simulink model "Simulink"  (R2024b)
settings: Solver=FixedStepAuto  StartTime=0.0  StopTime=tf_sim  FixedStep=dt/time_scale  MaxStep=dt/100  RelTol=1e-3
values from neighbouring files (symbols this model uses):
  A_ref = zeros(nx,nx,N_ref)    [Main.m]
  b_bar = repmat(b_tilde,N,1)    [Main.m]
  B_ref = zeros(nx,nu,N_ref)    [Main.m]
  d = 0.1    [Main.m]
  dt = tf_ref/N_ref    [Main.m]
  H_ter = terminalXf.H    [Main.m]
  h_ter = terminalXf.h    [Main.m]
  IC_obs = [IC_obs_state; IC_obs_d]    [Main.m]
  N = 20    [Main.m]
  nu = size(u_ref,2)    [Main.m]
  nx = size(x_ref,2)    [Main.m]
  Q_obs = blkdiag(Qw,Qp)    [Main.m]
  R_obs = diag([1 1 1])    [Main.m]
  time_scale = 1    [Main.m]
  Ub_lb = repmat(u_min,N_ref,1)-Umat2Uvect(u_ref)    [Main.m]
  Ub_ub = repmat(u_max,N_ref,1)-Umat2Uvect(u_ref)    [Main.m]
  v_max = 0.55    [Main.m]
  v_min = 0.2    [Main.m]
  w_max = 1    [Main.m]
  w_min = -1    [Main.m]
undefined symbols (not defined in the file or in its folder): Angular, DiscIntNeverNeededParam, H_sim, h_sim, Linear, S_sim, T_sim
libraries: robotlib x3
settings Model: Creator=nicvi  LastModifiedBy=vise
settings OptimizationCC: DefaultParameterBehavior=Inlined  EnhancedBackFolding=on  PassReuseOutputArgsAs=Individual arguments  ZeroExternalMemoryAtStartup=off  ZeroInternalMemoryAtStartup=off  MaxStackSize=64  OptimizeBlockOrder=speed  DifferentSizesBufferReuse=on  OptimizationCustomize=off  EfficientTunableParamExpr=on
settings DebuggingCC: ParameterTunabilityLossMsg=error
settings HardwareCC: ProdBitPerPointer=32  ProdBitPerSizeT=32  ProdBitPerPtrDiffT=32  ProdLargestAtomicFloat=None  ProdIntDivRoundTo=Undefined  ProdEndianess=Unspecified  ProdWordSize=32  ProdHWDeviceType=Generic->Unspecified (assume 32-bit Generic)  UseEmbeddedCoderFeatures=off
settings RTWCC: Description=Embedded Coder  SystemTargetFile=ert.tlc  HardwareBoard=Robot Operating System (ROS)  TLCOptions="-aInlineSetEventsForThisBaseRateFcn=TLC_FALSE -aSuppressMultiTaskScheduler=TLC_FALSE  -aRateBasedStepFcn=0"  TemplateMakefile=ert_default_tmf  Toolchain=Catkin  TargetLang=C++
settings CodeAppCC: ForceParamTrailComments=on  IgnoreCustomStorageClasses=off  OperatorAnnotations=on  SimulinkDataObjDesc=on  SFDataObjDesc=on  InsertBlockDesc=on
settings ERTTargetCC: SupportNonInlinedSFcns=on

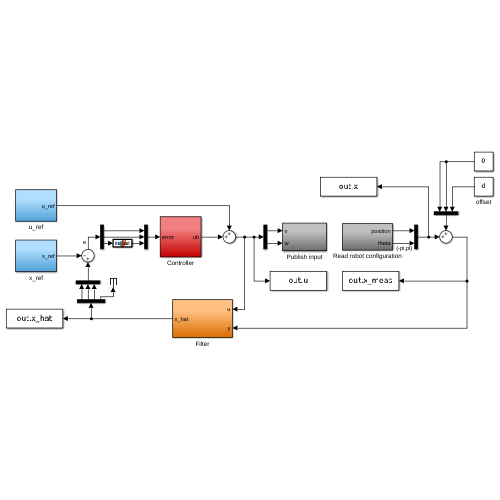
[thumbnail: Simulink's stored preview of the top-level diagram]
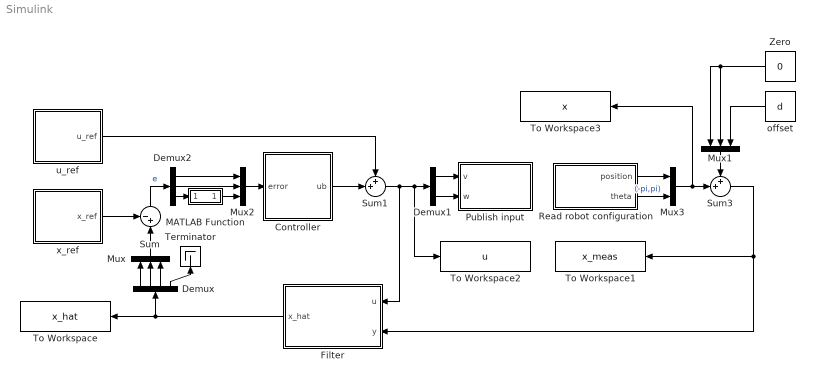
== system Simulink ==
  Controller : Subsystem
  Demux : Demux
  Demux1 : Demux  Outputs=2
  Demux2 : Demux  Outputs=3
  Filter : Subsystem
  MATLAB Function : MATLAB Function  TreatAsAtomicUnit=on
  Mux : Mux  Inputs=3
  Mux1 : Mux  Inputs=3
  Mux2 : Mux  Inputs=3
  Mux3 : Mux  Inputs=2
  Publish input : Subsystem
  Read robot configuration : Subsystem
  Sum : Sum  Inputs=-+|
  Sum1 : Sum  Inputs=++|
  Sum3 : Sum  Inputs=++|
  Terminator : Terminator
  To Workspace : ToWorkspace  VariableName=x_hat  SampleTime=-1
  To Workspace1 : ToWorkspace  VariableName=x_meas  SampleTime=-1
  To Workspace2 : ToWorkspace  VariableName=u  SampleTime=dt/time_scale
  To Workspace3 : ToWorkspace  VariableName=x  SampleTime=-1
  Zero : Constant  Value=0  OutDataTypeStr=Inherit: Inherit via back propagation
  offset : Constant  Value=d
  u_ref : Subsystem
  x_ref : Subsystem
  wires:
  x_ref/1(x_ref) -> Sum/1
  Controller/1(ub) -> Sum1/2
  u_ref/1(u_ref) -> Sum1/1
  Sum/1 -> Demux2/1  "e"
  Sum1/1 -> Filter/1(u), Demux1/1, To Workspace2/1
  Mux3/1 -> To Workspace3/1, Sum3/2
  Filter/1(x_hat) -> To Workspace/1, Demux/1
  Demux/1 -> Mux/1
  Demux/4 -> Terminator/1
  Demux/2 -> Mux/2
  Demux/3 -> Mux/3
  Mux/1 -> Sum/2
  offset/1 -> Mux1/3
  Mux1/1 -> Sum3/1
  Demux2/3 -> MATLAB Function/1(in)
  MATLAB Function/1(out) -> Mux2/3
  Demux2/1 -> Mux2/1
  Demux2/2 -> Mux2/2
  Mux2/1 -> Controller/1(error)
  Zero/1 -> Mux1/1, Mux1/2
  Demux1/1 -> Publish input/1(v)
  Demux1/2 -> Publish input/2(w)
  Read robot configuration/1(position) -> Mux3/1
  Read robot configuration/2(theta) -> Mux3/2  "(-pi,pi)"
  Sum3/1 -> Filter/2(y), To Workspace1/1

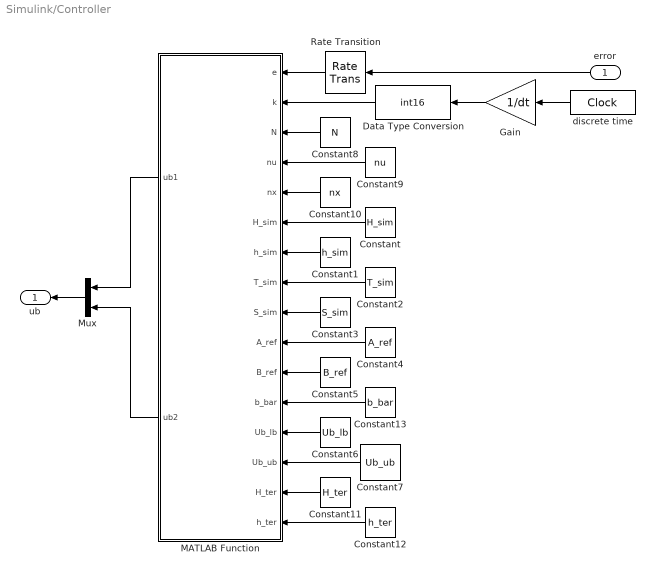
== system Simulink/Controller ==
  error : Inport
  Constant : Constant  Value=H_sim
  Constant1 : Constant  Value=h_sim
  Constant10 : Constant  Value=nx
  Constant11 : Constant  Value=H_ter
  Constant12 : Constant  Value=h_ter
  Constant13 : Constant  Value=b_bar
  Constant2 : Constant  Value=T_sim
  Constant3 : Constant  Value=S_sim
  Constant4 : Constant  Value=A_ref
  Constant5 : Constant  Value=B_ref
  Constant6 : Constant  Value=Ub_lb
  Constant7 : Constant  Value=Ub_ub
  Constant8 : Constant  Value=N
  Constant9 : Constant  Value=nu
  Data Type Conversion : DataTypeConversion  OutDataTypeStr=int16  SaturateOnIntegerOverflow=off  RndMeth=Floor
  Gain : Gain  Gain=1/dt
  MATLAB Function : MATLAB Function  TreatAsAtomicUnit=on
  Mux : Mux  Inputs=2
  Rate Transition : RateTransition  OutPortSampleTime=dt
  discrete time : DigitalClock  SampleTime=dt
  ub : Outport
  wires:
  Constant4/1 -> MATLAB Function/10(A_ref)
  Data Type Conversion/1 -> MATLAB Function/2(k)
  discrete time/1 -> Gain/1
  Gain/1 -> Data Type Conversion/1
  Rate Transition/1 -> MATLAB Function/1(e)
  Constant10/1 -> MATLAB Function/5(nx)
  Constant11/1 -> MATLAB Function/15(H_ter)
  Constant13/1 -> MATLAB Function/12(b_bar)
  Constant5/1 -> MATLAB Function/11(B_ref)
  Constant3/1 -> MATLAB Function/9(S_sim)
  Constant6/1 -> MATLAB Function/13(Ub_lb)
  Constant9/1 -> MATLAB Function/4(nu)
  Constant7/1 -> MATLAB Function/14(Ub_ub)
  Constant12/1 -> MATLAB Function/16(h_ter)
  Constant8/1 -> MATLAB Function/3(N)
  Constant1/1 -> MATLAB Function/7(h_sim)
  Constant2/1 -> MATLAB Function/8(T_sim)
  error/1 -> Rate Transition/1
  MATLAB Function/1(ub1) -> Mux/1
  MATLAB Function/2(ub2) -> Mux/2
  Mux/1 -> ub/1
  Constant/1 -> MATLAB Function/6(H_sim)

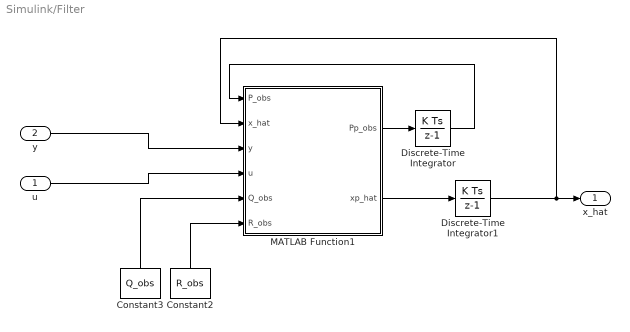
== system Simulink/Filter ==
  u : Inport
  y : Inport  Port=2
  Constant2 : Constant  Value=R_obs
  Constant3 : Constant  Value=Q_obs
  Discrete-Time Integrator : DiscreteIntegrator  InitialCondition=zeros(nx+1,nx+1)  SampleTime=-1  ICPrevOutput=DiscIntNeverNeededParam  ICPrevScaledInput=DiscIntNeverNeededParam
  Discrete-Time Integrator1 : DiscreteIntegrator  InitialCondition=IC_obs  SampleTime=-1  ICPrevOutput=DiscIntNeverNeededParam  ICPrevScaledInput=DiscIntNeverNeededParam
  MATLAB Function1 : MATLAB Function  TreatAsAtomicUnit=on
  x_hat : Outport
  wires:
  MATLAB Function1/1(Pp_obs) -> Discrete-Time Integrator/1
  Constant3/1 -> MATLAB Function1/5(Q_obs)
  Constant2/1 -> MATLAB Function1/6(R_obs)
  Discrete-Time Integrator/1 -> MATLAB Function1/1(P_obs)
  Discrete-Time Integrator1/1 -> x_hat/1, MATLAB Function1/2(x_hat)
  MATLAB Function1/2(xp_hat) -> Discrete-Time Integrator1/1
  y/1 -> MATLAB Function1/3(y)
  u/1 -> MATLAB Function1/4(u)

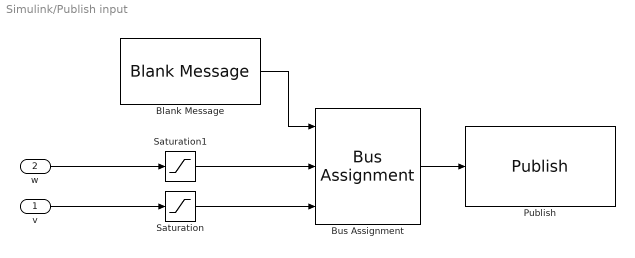
== system Simulink/Publish input ==
  v : Inport
  w : Inport  Port=2
  Blank Message : robotlib/Blank Message  messageClass=Message  entityType=geometry_msgs/Twist  messageType=geometry_msgs/Twist  SampleTime=dt  legacyBusStruct=off
  Bus Assignment : BusAssignment  AssignedSignals=Angular.Z,Linear.X
  Publish : robotlib/Publish  topicSource=Select from ROS network  topic=/cmd_vel  messageType=geometry_msgs/Twist  legacyBusStruct=off  messageQueueLength=1
  Saturation : Saturate  UpperLimit=v_max  LowerLimit=v_min
  Saturation1 : Saturate  UpperLimit=w_max  LowerLimit=w_min
  wires:
  Bus Assignment/1 -> Publish/1
  Blank Message/1 -> Bus Assignment/1
  w/1 -> Saturation1/1
  v/1 -> Saturation/1
  Saturation/1 -> Bus Assignment/3
  Saturation1/1 -> Bus Assignment/2

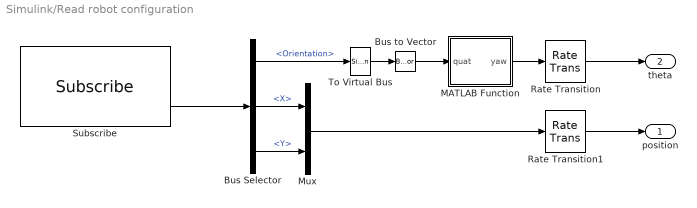
== system Simulink/Read robot configuration ==
  Bus Selector : BusSelector  OutputSignals=Pose.Pose.Orientation,Pose.Pose.Position.X,Pose.Pose.Position.Y
  Bus to Vector : BusToVector
  MATLAB Function : MATLAB Function  TreatAsAtomicUnit=on
  Mux : Mux  Inputs=2
  Rate Transition : RateTransition
  Rate Transition1 : RateTransition
  Subscribe : robotlib/Subscribe  topicSource=Select from ROS network  topic=/odom  messageType=nav_msgs/Odometry  SampleTime=dt  legacyBusStruct=off  messageQueueLength=1
  To Virtual Bus : SignalConversion  ConversionOutput=Virtual bus  OverrideOpt=off
  position : Outport
  theta : Outport  Port=2
  wires:
  Bus to Vector/1 -> MATLAB Function/1(quat)
  Bus Selector/1 -> To Virtual Bus/1  "<Orientation>"
  Bus Selector/2 -> Mux/1  "<X>"
  To Virtual Bus/1 -> Bus to Vector/1
  Subscribe/2 -> Bus Selector/1
  Bus Selector/3 -> Mux/2  "<Y>"
  MATLAB Function/1(yaw) -> Rate Transition/1
  Mux/1 -> Rate Transition1/1
  Rate Transition/1 -> theta/1
  Rate Transition1/1 -> position/1

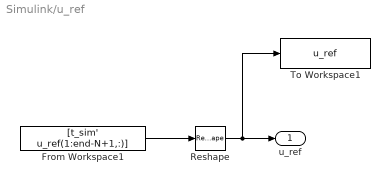
== system Simulink/u_ref ==
  From Workspace1 : FromWorkspace  VariableName="[t_sim'  u_ref(1:end-N+1,:)]"  SampleTime=dt
  Reshape : Reshape  OutputDimensionality=Column vector (2-D)
  To Workspace1 : ToWorkspace  VariableName=u_ref  SampleTime=dt/time_scale
  u_ref : Outport
  wires:
  From Workspace1/1 -> Reshape/1
  Reshape/1 -> To Workspace1/1, u_ref/1

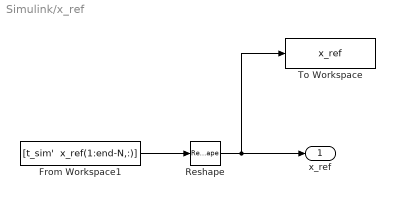
== system Simulink/x_ref ==
  From Workspace1 : FromWorkspace  VariableName="[t_sim'  x_ref(1:end-N,:)]"  SampleTime=dt
  Reshape : Reshape  OutputDimensionality=Column vector (2-D)
  To Workspace : ToWorkspace  VariableName=x_ref  SampleTime=dt/time_scale
  x_ref : Outport
  wires:
  From Workspace1/1 -> Reshape/1
  Reshape/1 -> To Workspace/1, x_ref/1

== matlab function Simulink/Controller/MATLAB Function ==
  data: e input; k input; ub1 output; N input; nu input; ub2 output; nx input; H_sim input; h_sim input; T_sim input; S_sim input; A_ref input; B_ref input; b_bar input; Ub_lb input; Ub_ub input; H_ter input; h_ter input
function [ub1,ub2]=MPC(e,k,N,nu,nx,H_sim,h_sim,T_sim,S_sim,A_ref,B_ref,b_bar,Ub_lb,Ub_ub,H_ter,h_ter)

k=k+1;
options=optimoptions('quadprog','Algorithm','active-set');

% Extract current matrices
H=H_sim(:,:,k);
h=h_sim(:,:,k);
T=T_sim(:,:,k);
S=S_sim(:,:,k);
A_ref_pred=A_ref(:,:,k:k+N-1);
B_ref_pred=B_ref(:,:,k:k+N-1);

% Generate constraints matrices
U_LB=Ub_lb((k-1)*nu+1:(k-1+N)*nu);  % estract lower bounds for ub in the current prediction horizon (input constraints)
U_UB=Ub_ub((k-1)*nu+1:(k-1+N)*nu);  % estract upper bounds for ub in the current prediction horizon (input constraints)
A_bar=zeros(2*N*nx,N*nx);                                                                     % generate matrices for inequality constraints ("state" (error) constraints)
B_bar=zeros(2*N*nx,N*nu);                                                                     % ...
for ii=1:N                                                                                    % ...
    A_bar(2*nx*(ii-1)+1:2*nx*ii,nx*(ii-1)+1:nx*ii)=[A_ref_pred(:,:,ii); -A_ref_pred(:,:,ii)]; % ...
    B_bar(2*nx*(ii-1)+1:2*nx*ii,nu*(ii-1)+1:nu*ii)=[B_ref_pred(:,:,ii); -B_ref_pred(:,:,ii)]; % ...
end                                                                                           % ...
A_ineq1=A_bar*S(1:end-nx,:)+B_bar;                                                            % ...
b_ineq1=b_bar-A_bar*T(1:end-nx,:)*e;                                                          % ...
A_ineq2=H_ter*S(end-nx+1:end,:);          % terminal constraint for the final error e(N) in the current horizon
b_ineq2=h_ter-H_ter*T(end-nx+1:end,:)*e;  % ...
A_ineq=[A_ineq1; A_ineq2];   % "total" inequality constraints
b_ineq=[b_ineq1; b_ineq2];   % ...

% quadprog solver for optimization
U0=(U_LB+U_UB)/2;
Ub_opt=quadprog(H,h*e,A_ineq,b_ineq,[],[],U_LB,U_UB,U0,options);

% Extract first control step
ub=Ub_opt(1:nu)';
ub1=ub(1);
ub2=ub(2);

end

== matlab function Simulink/Read robot configuration/MATLAB Function ==
  data: quat input; yaw output
function yaw=quat2yaw(quat)

q=zeros(1,4);

q(1)=quat(1);
q(2)=quat(2);
q(3)=quat(3);
q(4)=quat(4);

eul=quat2eul(q);

yaw=eul(3);

end

== matlab function Simulink/Filter/MATLAB Function1 ==
  data: P_obs input; Pp_obs output; x_hat input; y input; xp_hat output; u input; Q_obs input; R_obs input
function [Pp_obs,xp_hat]=EKF(P_obs,x_hat,y,u,Q_obs,R_obs)

nx=3;  % states
nw=2;  % input disturbance
nd=1;  % measurment offset

% Extended system model

f=@(x,u) [u(1)*cos(x(3));      % nonlinear extended model of the system - dynamics
          u(1)*sin(x(3));
               u(2)     
                0       ];  

h=@(x) [x(1) x(2) x(3)+x(4)]'; % nonlinear extended model of the system - output equation

% Linearisation around the extimated state

Aa=zeros(nx+nd,nx+nd);       % Aa = dfdx|x_hat,u
Aa(1,3)=-u(1)*sin(x_hat(3));
Aa(2,3)=u(1)*cos(x_hat(3));

Ca=[eye(nx) [0 0 1]'];       % Ca = dhdx|x_hat,u

La=zeros(nx+nd,nw+nd);       % La = dfdw|x_hat,u
La(1,1)=cos(x_hat(3));
La(2,1)=sin(x_hat(3));
La(3,2)=1;
La(4,3)=1;

Ma=eye(nx);                  % Ma = dhdn|x_hat,u

% Differential Riccati equation (P_obs is the (nx,nx) Riccati matrix)

Pp_obs=Aa*P_obs+P_obs*Aa'+La*Q_obs*La'-P_obs*Ca'*inv(Ma*R_obs*Ma')*Ca*P_obs;

% Kalman gain equation

K_obs=P_obs*Ca'*inv(R_obs);

% Filter equation

xp_hat=f(x_hat,u)+K_obs*(y-h(x_hat));

end

== matlab function Simulink/MATLAB Function ==
  data: in input; out output
function out = fcn(in)

out=mod(in+pi,2*pi)-pi;
